simulink model "Test_Tricopter_Model"  (R2015a)
settings: Solver=ode3  SolverMode=SingleTasking  StartTime=0.0  StopTime=20  FixedStep=T_sim  RelTol=1e-3
PreLoadFcn:
  | LoadLibraries
values from neighbouring files (symbols this model uses):
  a = 10.26    [SetupComplete.m]
  A_x = 0.015    [SetupComplete.m]
  A_y = A_x    (= 0.015)    [SetupComplete.m]
  A_z = 0.16    [SetupComplete.m]
  C_d0 = 0.001193    [SetupComplete.m]
  C_x = 1.2    [SetupComplete.m]
  C_y = C_x    (= 1.2)    [SetupComplete.m]
  C_z = 2.2    [SetupComplete.m]
  CG_0 = [0,0,0.02]'    [SetupComplete.m]
  g = 9.81    [SetupComplete.m]
  h = 0.08    [SetupComplete.m]
  h_FA = 0.02    [SetupComplete.m]
  h_M = 0.064    [SetupComplete.m]
  I_BAC_0 = [ Ix,0,Ixz;0,Iy,0;Ixz,0,Iz]    [SetupComplete.m]
  I_prop = 1/4*M_eq*R^2*diag([1,1,2])    [SetupComplete.m]
  I_tube = [1/2*M_tube*R_tube_eq^2,0,  0  ;           0 ,1/3*M_tube*l_arm^2,0;             0  ,0,1/3*M_tube*l_arm^2]    [SetupComplete.m]
  Initial_Omegas = [1;1;1]*Omega_hover    [Run3Copter.m]
  J_FA = I_prop(1,1) + m_prop*h^2  + m_FA*h_FA^2 + m_M*h_M^2    [SetupComplete.m]
  J_T = J_m+1/2*M_eq*R^2    (= 2.000642e-05)    [SetupComplete.m]
  Ki = lqi(LM_4DOF_aug, Q,R)    [robust_controller.m]
  l = 0.3450    (= 0.345)    [NDI_components.m]    (also in SetupComplete.m; robust_controller.m)
  l_arm = 0.264    [SetupComplete.m]
  m = 3.51    [SetupComplete.m]
  m_0 = 2.61    [SetupComplete.m]
  m_FA = 0.02    [SetupComplete.m]
  m_M = 0.300    (= 0.3)    [SetupComplete.m]
  m_prop = 0.02    [SetupComplete.m]
  R = 0.1778    [SetupComplete.m]    (also in robust_controller.m = eye(4))
  rho = 1.15    [SetupComplete.m]
  sigma = b*c/(pi*R)    (= 0.107416159567)    [SetupComplete.m]
  T_sim = 0.01    [Run3Copter.m]
  theta_0 = 0.38397    [SetupComplete.m]
  theta_1 = -0.2967    [SetupComplete.m]
  trim_simplemodel = [0.589627915568 -2.20656039197 0 0.588313336084 0 0 0.588313330414 0 0]    [trimvalues.mat]
  V_4DOF_last = [0.0122475086001 0.00870447045314 -0.0292257707267 -0.0198753669721 -0.00290766514824 -0.0269511839788 0.0344308792695 -0.0305235710433 -0.0274078219028 -0.0329291952852 -0.0272335702183 -0.00643013158961 ... (1500 elements, 50x30)]    [NN_c_weights.mat]
  v_i0 = sqrt( 1/3*m*g/(2*rho*pi*R^2)  )    [SetupComplete.m]
  W_4DOF_last = [0.0132359246225 -0.0402459595001 -0.0221501781133 0.0046881519205 0.0457506835434 0.0464888535199 -0.0342386918322 0.0470592781761 0.0457166948243 -0.00146243512772 0.0300280468889 -0.0358113661373 ... (204 elements, 4x51)]    [NN_c_weights.mat]
undefined symbols (not defined in the file or in its folder): DOWN_0, EAST_0, Motor, NORTH_0, P_0, Prop, Q_0, R_0, sigmatest, U_0, V_0, v_i_adim, Vx_adim, Vz_adim, W_0
undefined symbols (not defined in the file): Initial_Torques, Rotation_sign, Tau_motors
libraries: simulink x61, XXCopter x32, vrlib x26, simulink_extras x6, aerolib6dofsys x3, qcatlib x3, dspinverses x3, lib_controller x2, aerolibtransform2 x2, aerolib6dof2 x1
(part 3 of 10)

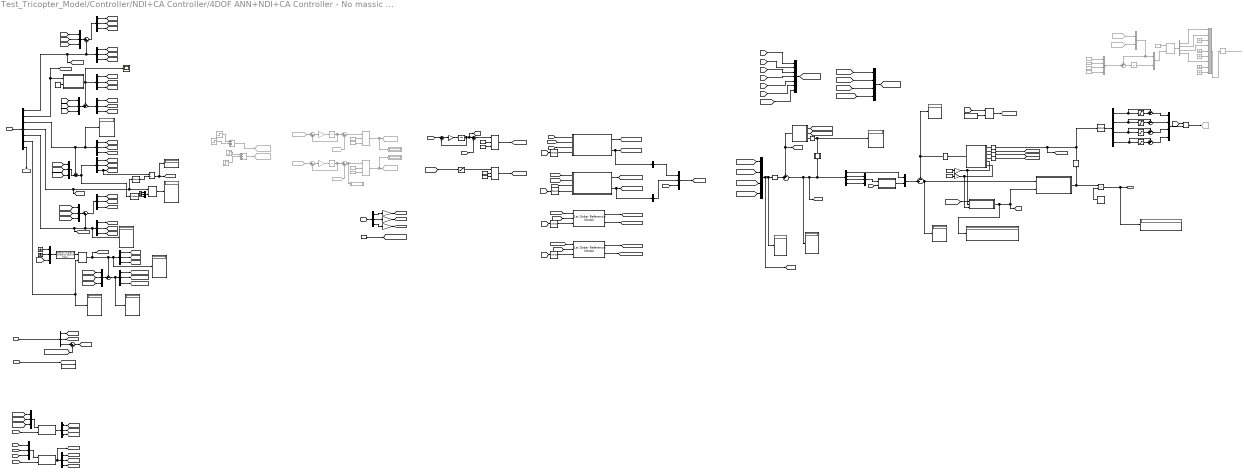
== system Test_Tricopter_Model/Controller/NDI+CA Controller/4DOF ANN+NDI+CA Controller - No massic update ==
  note: Gravity E2B
  note: ANN
  note: Rad2Deg
  note: Earth2Body
  note: ANN variables
  note: Input demux
  note: PCH
  note: Outer speed loop
  note: Speed references generator
  note: 0.26
  note: 19.5
  note: LQR test
  note: Roll and pitch angle provide X and Y acc in Earth axis (around hovering point). So requested increments in speed (error speed) will generate attitude commands
  note: Saturation block to avoid z_error going to
      |  infty when phi/theta -> 90deg
  note: Inner loop reference tuning / testing
  note: Earth <-> Body Angular Rate Conversions
  note: Reference generation for Rate Command Channels RCAH (for simulation purposes)
  note: ACAH for phi channel
  note: NDI 4DOF - WPQR
  note: Controller output:
      | 1. tau_1 [0-1] (Thr ottle motor 1)
      | 2. eta_1 (deg)  (Pan arm 1)
      | 3. gamma_1 (deg)  (Tilt arm 1)
      |
      | 4. tau_2 [0-1] (Throttle motor 2)
      | 5. eta_2 (deg)  (Pan arm 2)
      | 6. gamma_2 (deg)  (Tilt arm 2)
      |
      | 7. tau_3 [0-1] (Throttle motor 3)
      | 8. eta_3 (deg)  (Pan arm  3)
      | 9. gamma_3 (deg)  (Tilt arm 3)
  note: Throttle
  note: eta [deg]
  note: gamma[deg]
  note: eta1
  note: t3
  note: t2
  note: t1
  note: w
      | p
      | q
      | r
  note: ACAH for theta channel
  note: RCAH for psi channel
  note: RCAH for Vz_b channel
  note: Inner Model reference Command Generator
  measurements : Inport
  earth_ref : Inport  Port=2
  trim_control_input : Inport  Port=3
  Reference_attitude : Inport  Port=4
  1st Order Reference Model : lib_controller/1st Order Reference Model  tau=0.15  r=2
  1st Order Reference Model1 : lib_controller/1st Order Reference Model  tau=0.5  r=3
  Adaptive NN : Subsystem  Variant=on  VariantControl=Variant  OverrideUsingVariant=NN on AoA
      mask Display:
      | image(imread('ANN.png'))
      | 
      | 
      | port_label('input', 2, 'State vars')
      | port_label('input', 1, 'Channel vars')
      | port_label('input', 3, 'v prev')
      | 
      | port_label('output', 1, 'v_ad^')
  Add : Sum  Commented=on  Inputs=+-+
  Add1 : Sum  Commented=on  Inputs=+-+
  B_online : Display
  Bus Creator : BusCreator  Inputs=7
  Bus Creator1 : BusCreator
  Bus Selector1 : BusSelector  OutputSignals=y_c
  Bus Selector2 : BusSelector  OutputSignals=y_c
  Bus Selector : BusSelector  OutputSignals=euler,omega_b,X_e,DCM,V_b,V_e,A_b
  Constant : Constant  Value=0
  Constant1 : Constant  Value=2
  Constant10 : Constant  Commented=on  Value=10 * pi /180
  Constant11 : Constant  Value=4
  Constant12 : Constant  Commented=on  Value=0.2 * pi /180
  Constant2 : Constant  Value=0.2
  Constant20 : Constant  Commented=on  Value=-Ki
  Constant{21..24} (4 alike) : Constant  Commented=on  Value=0
  Constant3 : Constant  Value=0.1
  Constant7 : Constant  Value=0
  Constant8 : Constant  Commented=on  Value=-10 * pi /180
  Constant9 : Constant  Commented=on  Value=-0.2 * pi /180
  Control Allocation 4DOF : Subsystem  Variant=on  OverrideUsingVariant=Variant1
  Demux{,1..8,10..11,13..14,17} (14 alike) : Demux  Outputs=3
  Demux12 : Demux
  Demux15 : Demux
  Demux16 : Demux  Commented=on
  Display{,1..3,5..7} (7 alike) : Display
  Display10 : Display  Commented=on
  Display8 : Display  Commented=on
  Display9 : Display  Commented=on
  Divide : Product  Inputs=*/
  Earth to EarthPsi : Product  Multiplication=Matrix(*)
  Earth to body : Product  Multiplication=Matrix(*)
  Earth to body1 : Product  Multiplication=Matrix(*)
  Earth to body3 : Product  Commented=on  Multiplication=Matrix(*)
  F(X) : MATLAB Function  TreatAsAtomicUnit=on
  From67 : From  Commented=on  GotoTag=Vx_Earth
  From68 : From  Commented=on  GotoTag=Vx_Earth_ref
  From69 : From  Commented=on  GotoTag=Vy_Earth
  From70 : From  Commented=on  GotoTag=Vy_Earth_ref
  From82 : From  Commented=on  GotoTag=omega_b
  From83 : From  Commented=on  GotoTag=vz_b
  G(X) 4DOF_WPQR : MATLAB Function  TreatAsAtomicUnit=on
  Gain : Gain
  Gain1 : Gain
  Goto Tag Visibility : GotoTagVisibility  GotoTag=trimmed_input
  Goto61 : Goto  Commented=on  GotoTag=theta_ref
  Goto62 : Goto  Commented=on  GotoTag=phi_ref
  Goto63 : Goto  Commented=on  GotoTag=Vx_Earth_ref
  Goto64 : Goto  Commented=on  GotoTag=Vy_Earth_ref
  Goto85 : Goto  Commented=on  GotoTag=pch  TagVisibility=global
  Gravity : Constant  Value=[0;0;m*g]
  Ground{,1..3} (4 alike) : Ground
  Ground{9..13} (5 alike) : Ground  Commented=on
  Integrator1 : Integrator  Commented=on
  Integrator2 : Integrator  Commented=on
  Integrator3 : Integrator  Commented=on
  Integrator7 : Integrator
  Kq : Constant  Value=0.26
  Kref psi : Gain  Gain=6
  Kref psi1 : Gain  Gain=pi/180
  Kref psi2 : Gain  Gain=pi/180
  Kref psi4 : Gain  Gain=pi/180
  Kref vx : Gain  Commented=on  Gain=-3
  Kref vy : Gain  Commented=on  Gain=3
  Kt : Constant  Value=19.5
  Measurement noise : Subsystem  mask{sigma_noise=0.01*pi/180}
  Memory : Memory  X0=[0,0,0,0,0,0,0,0,0]  LinearizeAsDelay=on
  Memory1 : Memory
  Mux{,1..3,5..7,10..12,15} (11 alike) : Mux  Inputs=3
  Mux14 : Mux
  Mux18 : Mux  Commented=on  Inputs=2
  Mux19 : Mux  Commented=on  Inputs=2
  Mux20 : Mux  Commented=on  Inputs=9
  Mux21 : Mux  Commented=on
  Mux4 : Mux
  Mux8 : Mux  Inputs=2
  PID Controller1 : simulink/Continuous/PID Controller  Controller=PI  TimeDomain=Continuous-time  SampleTime=-1  IntegratorMethod=Forward Euler  FilterMethod=Forward Euler  Form=Parallel  UseFilter=on  ControllerParametersSource=external  P=1  I=1  D=0  N=100  InitialConditionSource=internal  InitialConditionForIntegrator=0  InitialConditionForFilter=0  ExternalReset=none  LimitOutput=off  UpperSaturationLimit=inf  LowerSaturationLimit=-inf  LinearizeAsGain=on  AntiWindupMode=none  Kb=1  TrackingMode=off  Kt=1  PParamMin=[]  PParamMax=[]  IParamMin=[]  IParamMax=[]  DParamMin=[]  DParamMax=[]  NParamMin=[]  NParamMax=[]  KbParamMin=[]  KbParamMax=[]  KtParamMin=[]  KtParamMax=[]  POutMin=[]  POutMax=[]  IOutMin=[]  IOutMax=[]  DOutMin=[]  DOutMax=[]  NOutMin=[]  NOutMax=[]  KbOutMin=[]  KbOutMax=[]  KtOutMin=[]  KtOutMax=[]  IntegratorOutMin=[]  IntegratorOutMax=[]  FilterOutMin=[]  FilterOutMax=[]  SumOutMin=[]  SumOutMax=[]  SumI1OutMin=[]  SumI1OutMax=[]  SumI2OutMin=[]  SumI2OutMax=[]  SumI3OutMin=[]  SumI3OutMax=[]  SumDOutMin=[]  SumDOutMax=[]  SaturationOutMin=[]  SaturationOutMax=[]  IntegratorContinuousStateAttributes=''  IntegratorStateMustResolveToSignalObject=off  IntegratorRTWStateStorageClass=Auto  FilterContinuousStateAttributes=''  FilterStateMustResolveToSignalObject=off  FilterRTWStateStorageClass=Auto  DifferentiatorICPrevScaledInput=0  DifferentiatorOutMin=[]  DifferentiatorOutMax=[]
  PID Controller2 : simulink/Continuous/PID Controller  Controller=PI  TimeDomain=Continuous-time  SampleTime=-1  IntegratorMethod=Forward Euler  FilterMethod=Forward Euler  Form=Parallel  UseFilter=on  ControllerParametersSource=external  P=1  I=1  D=0  N=100  InitialConditionSource=internal  InitialConditionForIntegrator=0  InitialConditionForFilter=0  ExternalReset=none  LimitOutput=off  UpperSaturationLimit=inf  LowerSaturationLimit=-inf  LinearizeAsGain=on  AntiWindupMode=none  Kb=1  TrackingMode=off  Kt=1  PParamMin=[]  PParamMax=[]  IParamMin=[]  IParamMax=[]  DParamMin=[]  DParamMax=[]  NParamMin=[]  NParamMax=[]  KbParamMin=[]  KbParamMax=[]  KtParamMin=[]  KtParamMax=[]  POutMin=[]  POutMax=[]  IOutMin=[]  IOutMax=[]  DOutMin=[]  DOutMax=[]  NOutMin=[]  NOutMax=[]  KbOutMin=[]  KbOutMax=[]  KtOutMin=[]  KtOutMax=[]  IntegratorOutMin=[]  IntegratorOutMax=[]  FilterOutMin=[]  FilterOutMax=[]  SumOutMin=[]  SumOutMax=[]  SumI1OutMin=[]  SumI1OutMax=[]  SumI2OutMin=[]  SumI2OutMax=[]  SumI3OutMin=[]  SumI3OutMax=[]  SumDOutMin=[]  SumDOutMax=[]  SaturationOutMin=[]  SaturationOutMax=[]  IntegratorContinuousStateAttributes=''  IntegratorStateMustResolveToSignalObject=off  IntegratorRTWStateStorageClass=Auto  FilterContinuousStateAttributes=''  FilterStateMustResolveToSignalObject=off  FilterRTWStateStorageClass=Auto  DifferentiatorICPrevScaledInput=0  DifferentiatorOutMin=[]  DifferentiatorOutMax=[]
  PID Controller3 : simulink/Continuous/PID Controller  Commented=on  Controller=PI  TimeDomain=Continuous-time  SampleTime=-1  IntegratorMethod=Forward Euler  FilterMethod=Forward Euler  Form=Parallel  UseFilter=on  ControllerParametersSource=external  P=1  I=1  D=0  N=100  InitialConditionSource=internal  InitialConditionForIntegrator=0  InitialConditionForFilter=0  ExternalReset=none  LimitOutput=off  UpperSaturationLimit=inf  LowerSaturationLimit=-inf  LinearizeAsGain=on  AntiWindupMode=none  Kb=1  TrackingMode=off  Kt=1  PParamMin=[]  PParamMax=[]  IParamMin=[]  IParamMax=[]  DParamMin=[]  DParamMax=[]  NParamMin=[]  NParamMax=[]  KbParamMin=[]  KbParamMax=[]  KtParamMin=[]  KtParamMax=[]  POutMin=[]  POutMax=[]  IOutMin=[]  IOutMax=[]  DOutMin=[]  DOutMax=[]  NOutMin=[]  NOutMax=[]  KbOutMin=[]  KbOutMax=[]  KtOutMin=[]  KtOutMax=[]  IntegratorOutMin=[]  IntegratorOutMax=[]  FilterOutMin=[]  FilterOutMax=[]  SumOutMin=[]  SumOutMax=[]  SumI1OutMin=[]  SumI1OutMax=[]  SumI2OutMin=[]  SumI2OutMax=[]  SumI3OutMin=[]  SumI3OutMax=[]  SumDOutMin=[]  SumDOutMax=[]  SaturationOutMin=[]  SaturationOutMax=[]  IntegratorContinuousStateAttributes=''  IntegratorStateMustResolveToSignalObject=off  IntegratorRTWStateStorageClass=Auto  FilterContinuousStateAttributes=''  FilterStateMustResolveToSignalObject=off  FilterRTWStateStorageClass=Auto  DifferentiatorICPrevScaledInput=0  DifferentiatorOutMin=[]  DifferentiatorOutMax=[]
  PID Controller4 : simulink/Continuous/PID Controller  Commented=on  Controller=PI  TimeDomain=Continuous-time  SampleTime=-1  IntegratorMethod=Forward Euler  FilterMethod=Forward Euler  Form=Parallel  UseFilter=on  ControllerParametersSource=external  P=1  I=1  D=0  N=100  InitialConditionSource=internal  InitialConditionForIntegrator=0  InitialConditionForFilter=0  ExternalReset=none  LimitOutput=off  UpperSaturationLimit=inf  LowerSaturationLimit=-inf  LinearizeAsGain=on  AntiWindupMode=none  Kb=1  TrackingMode=off  Kt=1  PParamMin=[]  PParamMax=[]  IParamMin=[]  IParamMax=[]  DParamMin=[]  DParamMax=[]  NParamMin=[]  NParamMax=[]  KbParamMin=[]  KbParamMax=[]  KtParamMin=[]  KtParamMax=[]  POutMin=[]  POutMax=[]  IOutMin=[]  IOutMax=[]  DOutMin=[]  DOutMax=[]  NOutMin=[]  NOutMax=[]  KbOutMin=[]  KbOutMax=[]  KtOutMin=[]  KtOutMax=[]  IntegratorOutMin=[]  IntegratorOutMax=[]  FilterOutMin=[]  FilterOutMax=[]  SumOutMin=[]  SumOutMax=[]  SumI1OutMin=[]  SumI1OutMax=[]  SumI2OutMin=[]  SumI2OutMax=[]  SumI3OutMin=[]  SumI3OutMax=[]  SumDOutMin=[]  SumDOutMax=[]  SaturationOutMin=[]  SaturationOutMax=[]  IntegratorContinuousStateAttributes=''  IntegratorStateMustResolveToSignalObject=off  IntegratorRTWStateStorageClass=Auto  FilterContinuousStateAttributes=''  FilterStateMustResolveToSignalObject=off  FilterRTWStateStorageClass=Auto  DifferentiatorICPrevScaledInput=0  DifferentiatorOutMin=[]  DifferentiatorOutMax=[]
  Phi Model Reference : Subsystem  mask{omega_n=4, xi=0.707, r=2}
      mask prompts: omega_n "Natural Frequency"; xi "Damping"; r "NN Error dynamic ratio"
      mask help:
      | 2nd Order Model Reference System
      | Natural frequency and damping ratio set the dynamic of the model reference.
      | Error dynamic ratio sets how faster compared to the reference model dynamics
      | is the settling time of the inversion error provided by the NN.
      mask Display:
      | TF = tf([omega_n^2],[1 2*xi*omega_n omega_n^2]);
      | 
      | [y,t]=step(TF);
      | S = stepinfo(y,t);
      | 
      | pos = get_param(gcb, 'Position');
      | width = pos(3) - pos(1);
      | height = pos(4) - pos(2);
      | t = t.*width/max(t);
      | y=y.*height/max(y);
      | plot(t,y);
      | S2 = stepinfo(y,t);
      | 
      | if S.Overshoot==0 % 1st order response
      |     text(S2.RiseTime ,height*0.85,['Rise time = ',num2str(S.RiseTime),'s' ]);
      |     text(S2.RiseTime ,height*0.75,['Settling Time = ',num2str(S.SettlingTime)]);
      | 
      | elseif S.Overshoot<0.05 % 2nd order response
      |     text(width*0.5 ,height*0.9,['Rise time = ',num2str(S.RiseTime),'s' ]);
      |     text(width*0.5 ,height*0.8,['Pike time = ',num2str(S.PeakTime),'s' ]);
      |     text(width*0.5 ,height*0.7,['Os = ',num2str(S.Peak)]);
      |     text(width*0.5 ,height*0.6,['SettlingTime = ',num2str(S.SettlingTime)]);
      | else % 2nd order response
      |     text(S2.PeakTime ,S2.Peak*0.85,['Peak time = ',num2str(S.PeakTime),'s' ]);
      |     text(S2.PeakTime ,S2.Peak*0.75,['Os = ',num2str(S.Peak)]);
      |     text(S2.PeakTime ,S2.Peak*0.65,['SettlingTime = ',num2str(S.SettlingTime)]);
      | end
      | 
      | 
      | [num,den] = tfdata(TF);
      | dpoly(num{:},den{:}, 's');
  Product : Product
  Product2 : Product  Multiplication=Matrix(*)
  Reshape : Reshape
  Reshape2 : Reshape  OutputDimensionality=Column vector (2-D)  OutputDimensions=[6,1]
  Reshape{3..6} (4 alike) : Reshape  OutputDimensions=[6,1]
  Reshape7 : Reshape  Commented=on  OutputDimensions=[6,1]
  Rotation Angles to Direction Cosine Matrix : aerolibtransform2/Rotation Angles to Direction Cosine Matrix  rotationOrder=ZYX
  Rotational Kinematics : MATLAB Function  TreatAsAtomicUnit=on
  Rotational Kinematics1 : MATLAB Function  TreatAsAtomicUnit=on
  Rotational Kinematics2 : MATLAB Function  TreatAsAtomicUnit=on
  Saturation : Saturate  UpperLimit=4  LowerLimit=-4
  Saturation1 : Saturate  UpperLimit=1  LowerLimit=0
  Saturation2 : Saturate  UpperLimit=deg2rad(160)  LowerLimit=-deg2rad(165)
  Saturation3 : Saturate  UpperLimit=1  LowerLimit=0
  Saturation4 : Saturate  UpperLimit=1  LowerLimit=0
  Scope1 : Scope
      settings: YMin=-2  YMax=2  SaveName=ScopeData15
  Selector : Selector  InputPortWidth=3  Indices=[3]
  Selector1 : Selector  NumberOfDimensions=2  InputPortWidth=[9]  IndexOptions=Index vector (dialog),Index vector (dialog)  Indices=3,3  OutputSizes=1,1
  Selector4 : Selector  InputPortWidth=9  Indices=[1 2 4 7]
  Selector5 : Selector  InputPortWidth=4  Indices=[2]
  Selector6 : Selector  InputPortWidth=4  Indices=[3]
  Selector7 : Selector  InputPortWidth=4  Indices=[4]
  Selector8 : Selector  InputPortWidth=4  Indices=[1]
  "Sigmoid " : Subsystem  mask{a=0.15}
      mask prompts: a "Sigmoid a param"
      mask TypeOptions a: a/Value
      mask Display:
      | x=-25:0.1:25;
      | 
      | y=(2.0 ./ (1.0 + exp(-a.*x))-1) ;
      | y2=zeros(size(x));
      | 
      | plot(x,y,x,y2);
      | 
      | %text(-20,0.5, ['a= ',num2str(a)])
  Step1 : Step  Commented=on  Time=5  After=5  SampleTime=0
  Step2 : Step  Commented=on  Time=10  After=5  SampleTime=0
  Step4 : Step  Commented=on  Time=5  After=5  SampleTime=0
  Step5 : Step  Commented=on  Time=10  After=10  SampleTime=0
  Sum{,4..5,25..26} (5 alike) : Sum  Inputs=|+-
  Sum{1..3,18..19,22,24,27..28} (9 alike) : Sum  Inputs=-+|
  Sum10 : Sum  Commented=on  Inputs=|+-
  Sum12 : Sum  Commented=on  Inputs=|+-
  Sum17 : Sum  Commented=on  Inputs=|+-
  Sum23 : Sum  Commented=on  Inputs=-+|
  Sum9 : Sum  Commented=on  Inputs=|++
  Theta Model Reference1 : Subsystem  mask{omega_n=4, xi=0.707, r=2}
      mask prompts: omega_n "Natural Frequency"; xi "Damping"; r "NN Error dynamic ratio"
      mask help:
      | 2nd Order Model Reference System
      | Natural frequency and damping ratio set the dynamic of the model reference.
      | Error dynamic ratio sets how faster compared to the reference model dynamics
      | is the settling time of the inversion error provided by the NN.
      mask Display:
      | TF = tf([omega_n^2],[1 2*xi*omega_n omega_n^2]);
      | 
      | [y,t]=step(TF);
      | S = stepinfo(y,t);
      | 
      | pos = get_param(gcb, 'Position');
      | width = pos(3) - pos(1);
      | height = pos(4) - pos(2);
      | t = t.*width/max(t);
      | y=y.*height/max(y);
      | plot(t,y);
      | S2 = stepinfo(y,t);
      | 
      | if S.Overshoot==0 % 1st order response
      |     text(S2.RiseTime ,height*0.85,['Rise time = ',num2str(S.RiseTime),'s' ]);
      |     text(S2.RiseTime ,height*0.75,['Settling Time = ',num2str(S.SettlingTime)]);
      | 
      | elseif S.Overshoot<0.05 % 2nd order response
      |     text(width*0.5 ,height*0.9,['Rise time = ',num2str(S.RiseTime),'s' ]);
      |     text(width*0.5 ,height*0.8,['Pike time = ',num2str(S.PeakTime),'s' ]);
      |     text(width*0.5 ,height*0.7,['Os = ',num2str(S.Peak)]);
      |     text(width*0.5 ,height*0.6,['SettlingTime = ',num2str(S.SettlingTime)]);
      | else % 2nd order response
      |     text(S2.PeakTime ,S2.Peak*0.85,['Peak time = ',num2str(S.PeakTime),'s' ]);
      |     text(S2.PeakTime ,S2.Peak*0.75,['Os = ',num2str(S.Peak)]);
      |     text(S2.PeakTime ,S2.Peak*0.65,['SettlingTime = ',num2str(S.SettlingTime)]);
      | end
      | 
      | 
      | [num,den] = tfdata(TF);
      | dpoly(num{:},den{:}, 's');
  Trimmed actuator signals{,2..5,7} (6 alike) : Display
  rad2deg : Constant  Value=[1, 180/pi, 0,1,0, 0, 1, 0,0]
  Controller output : Outport
  tag scope: attitude_com=global, trimmed_input=scoped, v_ad=global
  wires:
  earth_ref/1 -> Demux8/1
  Demux8/1 -> [Xearth_ref]
  Demux8/2 -> [Yearth_ref]
  Bus Selector/4 -> Earth to body/1, Selector1/1, [DCM]  "<DCM>"
  [Vz_body_ref] -> Mux3/3
  [Vx_body_ref] -> Mux3/1
  [Vy_body_ref] -> Mux3/2
  Demux6/3 -> [vz_error]
  Demux6/2 -> [vy_error]
  Demux6/1 -> [vx_error]
  Sum4/1 -> Demux6/1
  Bus Selector/5 -> [v_b], Sum4/2, Display2/1, Demux7/1  "<V_b>"
  Demux7/3 -> [vz_b]
  Demux7/2 -> [vy_b]
  Demux7/1 -> [vx_b]
  Mux3/1 -> Sum4/1
  [Zearth_ref] -> Mux1/3
  [Xearth_ref] -> Mux1/1
  [Yearth_ref] -> Mux1/2
  Mux1/1 -> Sum3/2
  Demux4/1 -> [Xe_error]
  Demux4/2 -> [Ye_error]
  Demux4/3 -> Divide/1, [Ze_error]
  Demux5/1 -> [X_earth]
  Demux5/2 -> [Y_earth]
  Demux5/3 -> [Z_earth]
  Bus Selector/3 -> Display/1, Demux5/1, Sum3/1  "<X_e>"
  [r_ref] -> Mux2/3
  [p_ref] -> Mux2/1
  [q_ref] -> Mux2/2
  Mux2/1 -> Sum1/2
  [psi_ref] -> Mux/3
  [phi_ref] -> Mux/1
  [theta_ref] -> Mux/2
  trim_control_input/1 -> [trimmed_input]
  Demux1/3 -> [psi_error]
  Demux1/2 -> [theta_error]
  Demux1/1 -> [phi_error]
  Demux/1 -> [p_error]
  Demux/2 -> [q_error]
  Demux/3 -> [r_error]
  Sum/1 -> Demux1/1
  Sum1/1 -> Demux/1
  Bus Selector/2 -> Measurement noise/1(Measurement), [omega_b]  "<omega_b>"
  Bus Selector/1 -> [att_Earth], Sum/2, Demux2/1  "<euler>"
  measurements/1 -> Bus Selector/1
  Demux2/3 -> [psi]
  Demux2/2 -> [theta]
  Demux2/1 -> [phi]
  Demux3/1 -> [p]
  Demux3/2 -> [q]
  Demux3/3 -> [r]
  Mux/1 -> Sum/1
  F(X)/1(fx) -> Reshape2/1
  [gforce_body] -> Reshape4/1  "gforce_body"
  Mux4/1 -> Trimmed actuator signals2/1, Reshape/1, [v_0]  "y_dot_desired"
  Reshape2/1 -> Sum2/1, Trimmed actuator signals7/1
  Reshape3/1 -> F(X)/1(prev_input)
  [omega_b] -> Reshape5/1  "omega_b"
  Reshape4/1 -> F(X)/2(gforce_body)
  Reshape5/1 -> F(X)/3(omega_body)
  Reshape6/1 -> F(X)/4(v_body)
  [v_b] -> Reshape6/1  "v_b"
  rad2deg/1 -> Product/2
  Memory/1 -> Selector4/1, [prev_output], Reshape3/1  "prev_output"
  Sum3/1 -> Demux4/1, Selector/1
  Sum2/1 -> Trimmed actuator signals4/1, Control Allocation 4DOF/1(Pseudocontrol input)  "y_dot_desired"
  [prev_output] -> G(X) 4DOF_WPQR/1(prev_input)
  [accZ_des] -> Mux4/1
  G(X) 4DOF_WPQR/1(gx) -> B_online/1, [gx], Control Allocation 4DOF/2(Effectiveness control matrix)
  Selector/1 -> Mux6/3
  Ground/1 -> Mux6/1
  Ground1/1 -> Mux6/2
  Mux6/1 -> Earth to body/2
  Earth to body/1 -> Display1/1
  Sum18/1 -> "Sigmoid "/1(In), Demux12/1, [v], Trimmed actuator signals3/1  "upsilon"
  Adaptive NN/1(v_ad^) -> Sum18/1, [v_ad]  "v_ad"
  "Sigmoid "/1(Out) -> Memory1/1, Trimmed actuator signals5/1
  Memory1/1 -> Adaptive NN/3(v_ad^ prev)
  [euler] -> Rotational Kinematics/2(Euler)
  Demux11/1 -> [p_ref]
  Demux11/2 -> [q_ref]
  Demux11/3 -> [r_ref]
  Rotational Kinematics/1(PQR) -> Demux11/1
  [phi_dot_ref] -> Mux11/1
  [theta_dot_ref] -> Mux11/2
  [psi_dot_ref] -> Mux11/3
  Mux11/1 -> Rotational Kinematics/1(Eulerdot)
  [euler] -> Rotational Kinematics1/2(Euler)
  Mux5/1 -> Rotational Kinematics1/1(PQR)
  [r] -> Mux5/3
  [p] -> Mux5/1
  [q] -> Mux5/2
  Demux10/1 -> [phi_dot]
  Demux10/2 -> [theta_dot]
  Demux10/3 -> [psi_dot]
  Rotational Kinematics1/1(Eulerdot) -> [euler_dot], Demux10/1
  Theta Model Reference1/1(y_dot_dot_des) -> [theta_dot_dot_desired]
  [phi_dot_dot_desired] -> Mux4/2
  [theta_dot_dot_desired] -> Mux4/3
  [psi_dot_dot_desired] -> Mux4/4
  Demux12/2 -> Mux7/1  "v_phi"
  Demux12/3 -> Mux7/2  "v_theta"
  Demux12/4 -> Mux7/3  "v_psi"
  Mux7/1 -> Rotational Kinematics2/1(Eulerdot)
  [euler] -> Rotational Kinematics2/2(Euler)
  Mux8/1 -> Sum2/2  "upsilon_b"
  Demux12/1 -> Mux8/1  "v_z"
  Rotational Kinematics2/1(PQR) -> Mux8/2  "upsilon_body"
  Integrator7/1 -> [psi_c], Sum26/1, Sum25/2  "psi_c"
  Kref psi/1 -> Integrator7/1
  Sum25/1 -> Kref psi/1
  [psi_ref] -> Sum25/1
  [psi] -> Sum26/2
  PID Controller1/1 -> [psi_dot_ref]  "psi_dot_ref"
  Constant1/1 -> PID Controller1/2
  Constant2/1 -> PID Controller1/3
  Sum26/1 -> PID Controller1/1  "psi_error"
  1st Order Reference Model1/1 -> [accZ_des]
  [Vz_body_ref] -> 1st Order Reference Model1/1
  Constant11/1 -> PID Controller2/2
  Constant3/1 -> PID Controller2/3
  [z_error] -> Saturation/1
  Selector1/1 -> Divide/2
  Divide/1 -> Display3/1, [z_error]
  [phi_ref] -> Phi Model Reference/1(u_ref)
  [phi_dot] -> Phi Model Reference/2(y_dot)
  [phi] -> Phi Model Reference/3(y)
  Phi Model Reference/1(y_dot_dot_des) -> [phi_dot_dot_desired]
  [theta_ref] -> Theta Model Reference1/1(u_ref)
  [theta_dot] -> Theta Model Reference1/2(y_dot)
  [theta] -> Theta Model Reference1/3(y)
  [psi_dot_ref] -> 1st Order Reference Model/1
  [psi_dot] -> 1st Order Reference Model/2
  1st Order Reference Model/1 -> [psi_dot_dot_desired]
  [vz_b] -> 1st Order Reference Model1/2
  Phi Model Reference/2(NN_variables) -> Bus Selector1/1, [phi_channel_var]
  1st Order Reference Model1/2 -> [Vz_body__channel_var]
  1st Order Reference Model/2 -> [psi_channel_var]
  Theta Model Reference1/2(NN_variables) -> Bus Selector2/1, [theta_channel_var]
  [p] -> Bus Creator/3  "p"
  [theta] -> Bus Creator/2  "theta"
  [q] -> Bus Creator/4  "q"
  [phi] -> Bus Creator/1  "phi"
  [r] -> Bus Creator/5  "r"
  Bus Creator/1 -> [State_NN_Variables]
  [State_NN_Variables] -> Adaptive NN/2(System State Vars)
  [Vz_body__channel_var] -> Bus Creator1/4  "vertical acc channel"
  [psi_channel_var] -> Bus Creator1/3  "yaw channel"
  [theta_channel_var] -> Bus Creator1/2  "pitch channel"
  [phi_channel_var] -> Bus Creator1/1  "roll channel"
  Bus Creator1/1 -> [Channel_NN_Variables]
  [Channel_NN_Variables] -> Adaptive NN/1(Model Reference Vars)
  [prev_output] -> Bus Creator/7  "prev_outputs"
  [w] -> Bus Creator/6  "w"
  Demux17/1 -> Kref psi1/1
  Demux17/3 -> Kref psi4/1
  Kref psi1/1 -> [phi_ref]
  Kref psi2/1 -> [theta_ref]
  Kref psi4/1 -> [psi_ref]
  Demux8/3 -> Sum5/1
  Sum5/1 -> [Zearth_ref]
  Constant7/1 -> [Inc_Z_earth_reference]
  [Inc_Z_earth_reference] -> Sum5/2
  PID Controller2/1 -> [Vz_body_ref]
  Integrator1/1 -> Sum10/1, Sum9/2  "vx_c"
  Kref vx/1 -> Integrator1/1
  Sum9/1 -> Kref vx/1
  From68/1 -> Sum9/1
  From67/1 -> Sum10/2
  Constant8/1 -> PID Controller3/2
  Constant9/1 -> PID Controller3/3
  Sum10/1 -> PID Controller3/1  "vx_error"
  Integrator2/1 -> Sum17/1, Sum12/2  "vy_c"
  Kref vy/1 -> Integrator2/1
  Sum12/1 -> Kref vy/1
  From70/1 -> Sum12/1
  From69/1 -> Sum17/2
  Constant10/1 -> PID Controller4/2
  Constant12/1 -> PID Controller4/3
  Sum17/1 -> Display10/1, PID Controller4/1  "vy_error"
  Add/1 -> Goto63/1
  Add1/1 -> Goto64/1
  Saturation/1 -> PID Controller2/1
  [Vz_Earth_ref] -> Mux10/3
  [Vx_Earth_ref] -> Mux10/1
  [Vy_Earth_ref] -> Mux10/2
  Demux13/3 -> [Vz_Earth_error]
  Demux13/2 -> [Vy_Earth_error]
  Demux13/1 -> [Vx_Earth_error]
  Sum19/1 -> Display6/1, Demux13/1
  Bus Selector/6 -> Earth to EarthPsi/2, Display5/1  "<V_e>"
  Demux14/3 -> [Vz_Earth]
  Demux14/2 -> [Vy_Earth]
  Demux14/1 -> [Vx_Earth]
  Ground3/1 -> Mux12/1
  Ground2/1 -> Mux12/2
  [psi] -> Mux12/3
  Mux12/1 -> Rotation Angles to Direction Cosine Matrix/1
  Rotation Angles to Direction Cosine Matrix/1 -> Earth to EarthPsi/1
  Mux10/1 -> Sum19/2
  Earth to EarthPsi/1 -> Sum19/1, Display7/1, Demux14/1, [V_Earth]
  PID Controller3/1 -> Display8/1, Goto61/1  "theta_ref"
  PID Controller4/1 -> Display9/1, Goto62/1  "phi_ref"
  Bus Selector/7 -> [acc_b]  "<A_b>"
  Product/1 -> Controller output/1, Trimmed actuator signals/1
  Sum23/1 -> Integrator3/1
  From83/1 -> Mux18/1
  From82/1 -> Mux18/2
  Mux19/1 -> Earth to body3/2
  Mux18/1 -> Mux19/1, Sum23/1
  Integrator3/1 -> Mux19/2
  Mux20/1 -> Reshape7/1
  Ground9/1 -> Mux20/3
  Ground10/1 -> Mux20/5
  Ground11/1 -> Mux20/6
  Ground12/1 -> Mux20/8
  Ground13/1 -> Mux20/9
  Constant20/1 -> Earth to body3/1
  Earth to body3/1 -> Demux16/1
  Demux16/1 -> Mux20/1
  Demux16/2 -> Mux20/2
  Demux16/3 -> Mux20/4
  Demux16/4 -> Mux20/7
  Mux21/1 -> Sum23/2
  Constant24/1 -> Mux21/4
  Constant23/1 -> Mux21/3
  Constant22/1 -> Mux21/2
  Constant21/1 -> Mux21/1
  Reshape7/1 -> ?
  Reference_attitude/1 -> Demux17/1
  Demux17/2 -> Kref psi2/1
  Control Allocation 4DOF/1(Control output) -> Product/1, Memory/1
  Selector4/1 -> Demux15/1
  Saturation1/1 -> Sum22/2
  Demux15/1 -> Sum22/1, Saturation1/1
  Saturation2/1 -> Sum24/2
  Demux15/2 -> Sum24/1, Saturation2/1
  Saturation3/1 -> Sum27/2
  Demux15/3 -> Saturation3/1, Sum27/1
  Saturation4/1 -> Sum28/2
  Demux15/4 -> Saturation4/1, Sum28/1
  Sum22/1 -> Mux14/1
  Sum24/1 -> Mux14/2
  Sum27/1 -> Mux14/3
  Sum28/1 -> Mux14/4
  Mux14/1 -> Product2/2
  [gx] -> Product2/1
  [pch] -> Selector5/1
  [pch] -> Selector6/1
  [pch] -> Selector7/1
  Selector7/1 -> 1st Order Reference Model/3
  Selector8/1 -> 1st Order Reference Model1/3
  [pch] -> Selector8/1
  Bus Selector2/1 -> Mux15/2  "<y_c>"
  Bus Selector1/1 -> Mux15/1  "<y_c>"
  Mux15/1 -> [attitude_com]  "attitude_com"
  Measurement noise/1(Noisy Output) -> Scope1/1, Demux3/1, Sum1/1
  Constant/1 -> Measurement noise/2(Activate)
  Selector5/1 -> Phi Model Reference/4(pch)
  Selector6/1 -> Theta Model Reference1/4(pch)
  Reshape/1 -> Sum18/2  "upsilon"
  Kt/1 -> Gain/1
  Step1/1 -> Add/1
  Step2/1 -> Add/2
  Step4/1 -> Add1/1
  Step5/1 -> Add1/2
  Gain/1 -> G(X) 4DOF_WPQR/2(Kt), F(X)/5(Kt)
  Kq/1 -> Gain1/1
  Gain1/1 -> G(X) 4DOF_WPQR/3(Kq), F(X)/6(Kq)
  [psi_c] -> Mux15/3
  Gravity/1 -> Earth to body1/2
  Earth to body1/1 -> [gforce_body]
  [DCM] -> Earth to body1/1
  Product2/1 -> Goto85/1  "pch"
